simulink model "C_H_B - Copy"  (R2017a)
settings: Solver=ode23t  StartTime=0.0  StopTime=0.08  FixedStep=5e-5  MaxStep=1e-4  RelTol=1e-3
undefined symbols (not defined in the file): a1, a2, a3, Vdc
libraries: powerlib x50, simulink x6
settings Model: Creator=Vinay  LastModifiedBy=murra

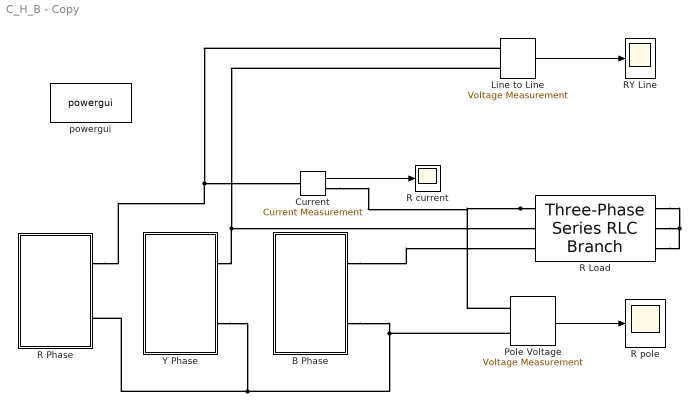
== system C_H_B - Copy ==
  B Phase : Subsystem
  Current : powerlib/Measurements/Current Measurement  PhasorSimulation=off  OutputType=Complex  PSBequivalent=0
  Line to Line : powerlib/Measurements/Voltage Measurement  PhasorSimulation=off  OutputType=Complex  PSBequivalent=0
  "Pole Voltage  " : powerlib/Measurements/Voltage Measurement  PhasorSimulation=off  OutputType=Complex  PSBequivalent=0
  R Load : powerlib/Elements/Three-Phase Series RLC Branch  LConnTagsString=A|B|C  RConnTagsString=A|B|C  BranchType=RL  Resistance=100  Inductance=1.5e-3  Capacitance=1e-6  Measurements=None
  R Phase : Subsystem
  R current : Scope
  R pole : Scope
  RY Line : Scope
  Y Phase : Subsystem
  powergui : powerlib/powergui  Priority=1  SimulationMode=Discrete  SampleTime=1e-06  frequency=60  Iterations=50  frequencyindice=0  Pbase=100e6  ErrMax=1e-4  UnitsV=kV  UnitsW=MW  buscounter=0  FunctionMessages=off  echomessages=off  EnableUseOfTLC=off  CurrentSourceSwitches=off  DisableSnubberDevices=off  DisableRonSwitches=off  DisableVfSwitches=off  DisplayEquations=off  SolverType=Tustin/Backward Euler (TBE)  Interpol=off  ExternalGateDelay=off  methode=off  Ts=100  x0status=blocks  SPID=on  SwTol=0  HookPort=off  RestoreLinks=warning  ResistiveCurrentMeasurement=off  Frange=[0:2:500]  Ylog=off  Xlog=on  ShowGrid=off  save=off  variable=ZData  structure=Rpole  ZoomFFT=off  StartTime=0.02  cycles=2  DisplayStyle=2  fundamental=50  FreqAxis=off  MaxFrequency=10000  frequencyindicesteady=1  RmsSteady=1  display=off
  wires:
  Line to Line/1 -> RY Line/1
  "Pole Voltage  "/1 -> R pole/1
  Current/1 -> R current/1
  connections:
  B Phase/RConn2 -- "Pole Voltage  "/LConn2 -- Y Phase/RConn2 -- R Phase/RConn2
  R Phase/RConn1 -- Line to Line/LConn1 -- Current/LConn1
  Y Phase/RConn1 -- Line to Line/LConn2 -- R Load/LConn2
  B Phase/RConn1 -- R Load/LConn3
  R Load/RConn3 -- R Load/RConn1 -- R Load/RConn2
  R Load/LConn1 -- "Pole Voltage  "/LConn1 -- Current/RConn1

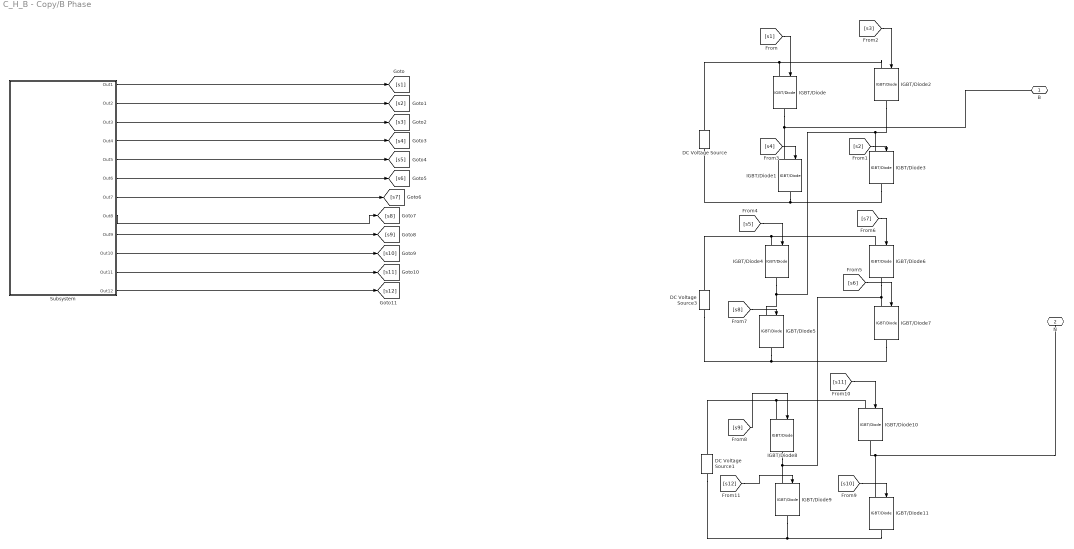
== system C_H_B - Copy/B Phase ==
  DC Voltage Source : powerlib/Electrical Sources/DC Voltage Source  Amplitude=Vdc  Measurements=None
  DC Voltage Source1 : powerlib/Electrical Sources/DC Voltage Source  Amplitude=Vdc  Measurements=None
  DC Voltage Source3 : powerlib/Electrical Sources/DC Voltage Source  Amplitude=Vdc  Measurements=None
  IGBT/Diode{,1..11} (12 alike) : powerlib/Power Electronics/IGBT//Diode  Ron=1e-3  Rs=1e5  Cs=inf  Measurements=off
  Subsystem : Subsystem
  B : PMIOPort  Port=1  Side=Right
  N : PMIOPort  Port=2  Side=Right
  wires:
  [s3] -> IGBT/Diode2/1
  [s6] -> IGBT/Diode7/1
  [s4] -> IGBT/Diode1/1
  [s8] -> IGBT/Diode5/1
  [s12] -> IGBT/Diode9/1
  [s2] -> IGBT/Diode3/1
  [s7] -> IGBT/Diode6/1
  [s9] -> IGBT/Diode8/1
  [s1] -> IGBT/Diode/1
  [s10] -> IGBT/Diode11/1
  [s5] -> IGBT/Diode4/1
  [s11] -> IGBT/Diode10/1
  Subsystem/5(Out5) -> [s5]
  Subsystem/7(Out7) -> [s7]
  Subsystem/8(Out8) -> [s8]
  Subsystem/3(Out3) -> [s3]
  Subsystem/10(Out10) -> [s10]
  Subsystem/1(Out1) -> [s1]
  Subsystem/11(Out11) -> [s11]
  Subsystem/2(Out2) -> [s2]
  Subsystem/12(Out12) -> [s12]
  Subsystem/6(Out6) -> [s6]
  Subsystem/9(Out9) -> [s9]
  Subsystem/4(Out4) -> [s4]
  connections:
  IGBT/Diode10/RConn1 -- IGBT/Diode11/LConn1 -- N/RConn1
  DC Voltage Source1/LConn1 -- IGBT/Diode11/RConn1 -- IGBT/Diode9/RConn1
  DC Voltage Source3/RConn1 -- IGBT/Diode6/LConn1 -- IGBT/Diode4/LConn1
  DC Voltage Source1/RConn1 -- IGBT/Diode10/LConn1 -- IGBT/Diode8/LConn1
  DC Voltage Source/RConn1 -- IGBT/Diode2/LConn1 -- IGBT/Diode/LConn1
  DC Voltage Source3/LConn1 -- IGBT/Diode7/RConn1 -- IGBT/Diode5/RConn1
  IGBT/Diode/RConn1 -- IGBT/Diode1/LConn1 -- B/RConn1
  IGBT/Diode9/LConn1 -- IGBT/Diode8/RConn1 -- IGBT/Diode7/LConn1 -- IGBT/Diode6/RConn1
  IGBT/Diode3/LConn1 -- IGBT/Diode2/RConn1 -- IGBT/Diode5/LConn1 -- IGBT/Diode4/RConn1
  DC Voltage Source/LConn1 -- IGBT/Diode1/RConn1 -- IGBT/Diode3/RConn1

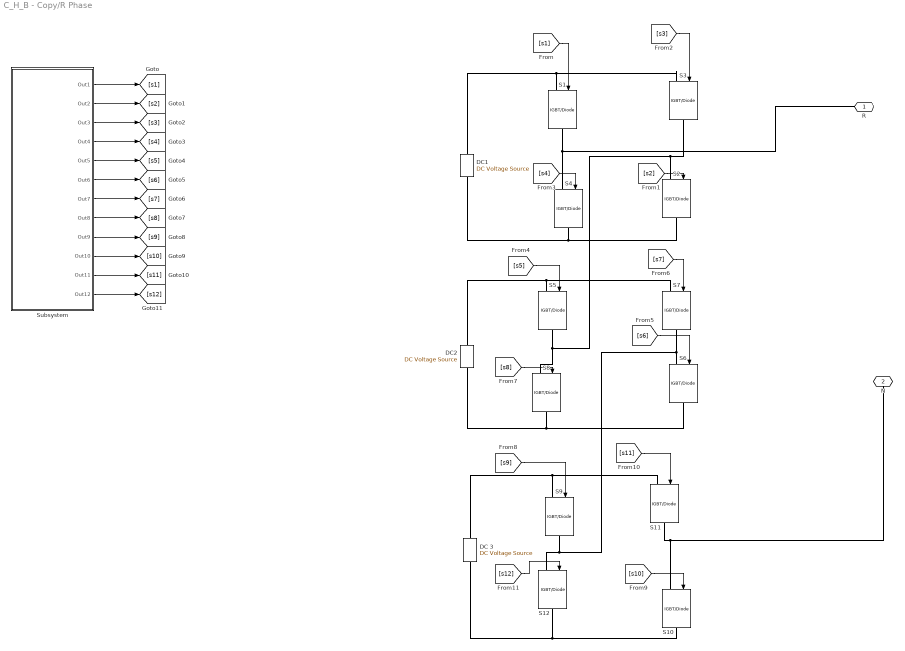
== system C_H_B - Copy/R Phase ==
  DC 3 : powerlib/Electrical Sources/DC Voltage Source  Amplitude=Vdc  Measurements=None
  DC1 : powerlib/Electrical Sources/DC Voltage Source  Amplitude=Vdc  Measurements=None
  DC2 : powerlib/Electrical Sources/DC Voltage Source  Amplitude=Vdc  Measurements=None
  S{1..12} (12 alike) : powerlib/Power Electronics/IGBT//Diode  Ron=1e-3  Rs=1e5  Cs=inf  Measurements=off
  Subsystem : Subsystem
  R : PMIOPort  Port=1  Side=Right
  N : PMIOPort  Port=2  Side=Right
  wires:
  [s3] -> S3/1
  [s6] -> S6/1
  [s4] -> S4/1
  [s8] -> S8/1
  [s12] -> S12/1
  [s2] -> S2/1
  [s7] -> S7/1
  [s9] -> S9/1
  [s1] -> S1/1
  [s10] -> S10/1
  [s5] -> S5/1
  [s11] -> S11/1
  Subsystem/5(Out5) -> [s5]
  Subsystem/7(Out7) -> [s7]
  Subsystem/8(Out8) -> [s8]
  Subsystem/3(Out3) -> [s3]
  Subsystem/10(Out10) -> [s10]
  Subsystem/1(Out1) -> [s1]
  Subsystem/11(Out11) -> [s11]
  Subsystem/2(Out2) -> [s2]
  Subsystem/12(Out12) -> [s12]
  Subsystem/6(Out6) -> [s6]
  Subsystem/9(Out9) -> [s9]
  Subsystem/4(Out4) -> [s4]
  connections:
  S11/RConn1 -- N/RConn1 -- S10/LConn1
  DC 3/LConn1 -- S10/RConn1 -- S12/RConn1
  DC2/RConn1 -- S7/LConn1 -- S5/LConn1
  DC 3/RConn1 -- S11/LConn1 -- S9/LConn1
  DC1/RConn1 -- S3/LConn1 -- S1/LConn1
  DC2/LConn1 -- S6/RConn1 -- S8/RConn1
  S1/RConn1 -- R/RConn1 -- S4/LConn1
  S12/LConn1 -- S9/RConn1 -- S6/LConn1 -- S7/RConn1
  S2/LConn1 -- S3/RConn1 -- S8/LConn1 -- S5/RConn1
  DC1/LConn1 -- S4/RConn1 -- S2/RConn1

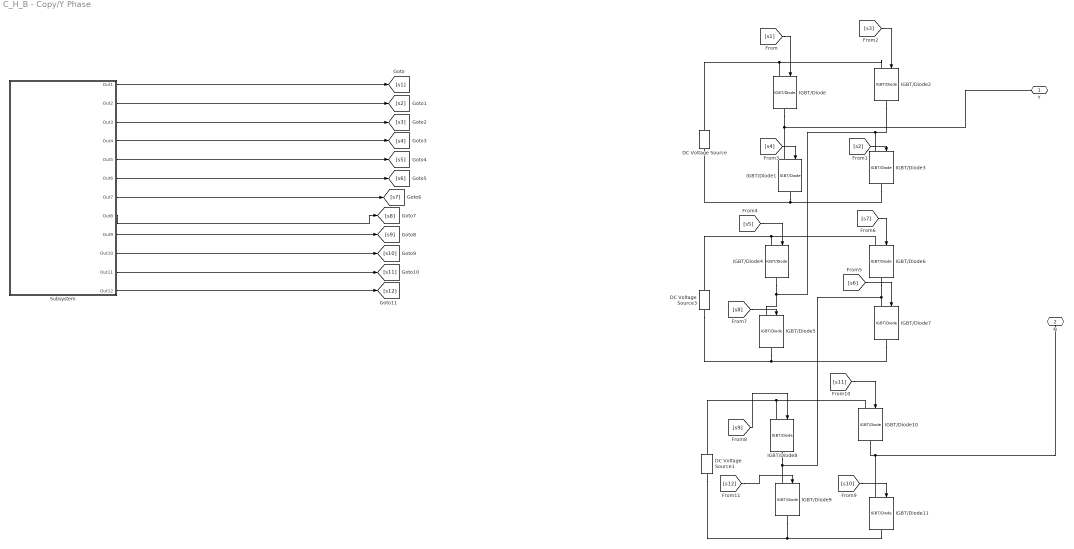
== system C_H_B - Copy/Y Phase ==
  DC Voltage Source : powerlib/Electrical Sources/DC Voltage Source  Amplitude=Vdc  Measurements=None
  DC Voltage Source1 : powerlib/Electrical Sources/DC Voltage Source  Amplitude=Vdc  Measurements=None
  DC Voltage Source3 : powerlib/Electrical Sources/DC Voltage Source  Amplitude=Vdc  Measurements=None
  IGBT/Diode{,1..11} (12 alike) : powerlib/Power Electronics/IGBT//Diode  Ron=1e-3  Rs=1e5  Cs=inf  Measurements=off
  Subsystem : Subsystem
  Y : PMIOPort  Port=1  Side=Right
  N : PMIOPort  Port=2  Side=Right
  wires:
  [s3] -> IGBT/Diode2/1
  [s6] -> IGBT/Diode7/1
  [s4] -> IGBT/Diode1/1
  [s8] -> IGBT/Diode5/1
  [s12] -> IGBT/Diode9/1
  [s2] -> IGBT/Diode3/1
  [s7] -> IGBT/Diode6/1
  [s9] -> IGBT/Diode8/1
  [s1] -> IGBT/Diode/1
  [s10] -> IGBT/Diode11/1
  [s5] -> IGBT/Diode4/1
  [s11] -> IGBT/Diode10/1
  Subsystem/5(Out5) -> [s5]
  Subsystem/7(Out7) -> [s7]
  Subsystem/8(Out8) -> [s8]
  Subsystem/3(Out3) -> [s3]
  Subsystem/10(Out10) -> [s10]
  Subsystem/1(Out1) -> [s1]
  Subsystem/11(Out11) -> [s11]
  Subsystem/2(Out2) -> [s2]
  Subsystem/12(Out12) -> [s12]
  Subsystem/6(Out6) -> [s6]
  Subsystem/9(Out9) -> [s9]
  Subsystem/4(Out4) -> [s4]
  connections:
  IGBT/Diode10/RConn1 -- IGBT/Diode11/LConn1 -- N/RConn1
  DC Voltage Source1/LConn1 -- IGBT/Diode11/RConn1 -- IGBT/Diode9/RConn1
  DC Voltage Source3/RConn1 -- IGBT/Diode6/LConn1 -- IGBT/Diode4/LConn1
  DC Voltage Source1/RConn1 -- IGBT/Diode10/LConn1 -- IGBT/Diode8/LConn1
  DC Voltage Source/RConn1 -- IGBT/Diode2/LConn1 -- IGBT/Diode/LConn1
  DC Voltage Source3/LConn1 -- IGBT/Diode7/RConn1 -- IGBT/Diode5/RConn1
  IGBT/Diode/RConn1 -- IGBT/Diode1/LConn1 -- Y/RConn1
  IGBT/Diode9/LConn1 -- IGBT/Diode8/RConn1 -- IGBT/Diode7/LConn1 -- IGBT/Diode6/RConn1
  IGBT/Diode3/LConn1 -- IGBT/Diode2/RConn1 -- IGBT/Diode5/LConn1 -- IGBT/Diode4/RConn1
  DC Voltage Source/LConn1 -- IGBT/Diode1/RConn1 -- IGBT/Diode3/RConn1

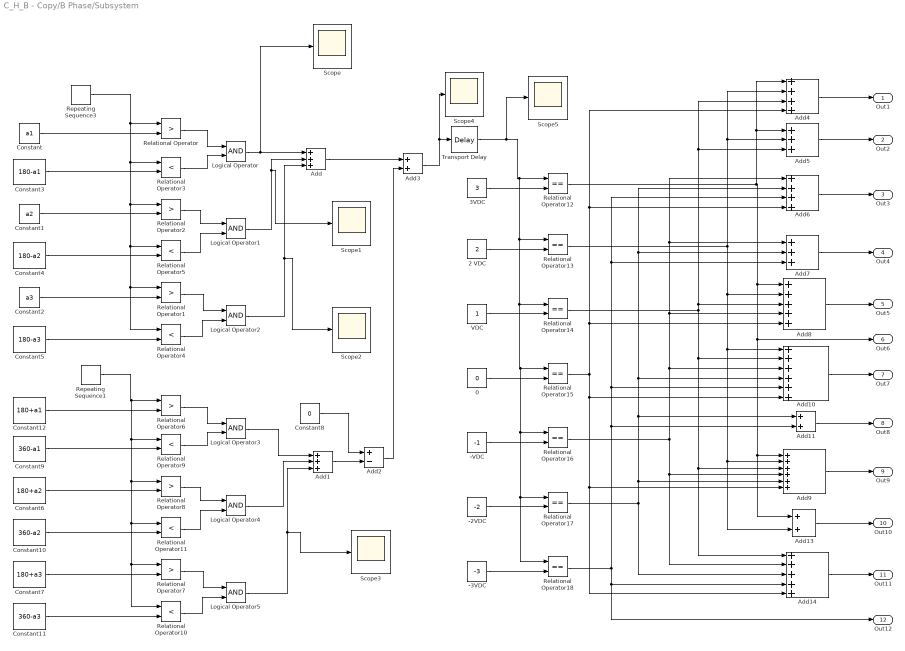
== system C_H_B - Copy/B Phase/Subsystem ==
  -2VDC : Constant  Value=-2
  -3VDC : Constant  Value=-3
  -VDC : Constant  Value=-1
  0 : Constant  Value=0
  2 VDC : Constant  Value=2
  3VDC : Constant  Value=3
  Add{,1,5,7} (4 alike) : Sum  Inputs=+++
  Add10 : Sum  Inputs=++++++
  Add11 : Sum
  Add13 : Sum
  Add14 : Sum  Inputs=+++++
  Add2 : Sum  Inputs=+-
  Add3 : Sum
  Add4 : Sum  Inputs=++++
  Add6 : Sum  Inputs=++++
  Add8 : Sum  Inputs=+++++
  Add9 : Sum  Inputs=++++++
  Constant : Constant  Value=a1
  Constant1 : Constant  Value=a2
  Constant10 : Constant  Value=360-a2
  Constant11 : Constant  Value=360-a3
  Constant12 : Constant  Value=180+a1
  Constant2 : Constant  Value=a3
  Constant3 : Constant  Value=180-a1
  Constant4 : Constant  Value=180-a2
  Constant5 : Constant  Value=180-a3
  Constant6 : Constant  Value=180+a2
  Constant7 : Constant  Value=180+a3
  Constant8 : Constant  Value=0
  Constant9 : Constant  Value=360-a1
  Logical Operator{,1..5} (6 alike) : Logic  AllPortsSameDT=off  OutDataTypeStr=boolean
  Relational Operator{,1..2,6..8} (6 alike) : RelationalOperator  Operator=>  OutDataTypeStr=boolean  RndMeth=Simplest
  Relational Operator{3..5,9..11} (6 alike) : RelationalOperator  Operator=<  OutDataTypeStr=boolean  RndMeth=Simplest
  Relational Operator{12..18} (7 alike) : RelationalOperator  Operator===  OutDataTypeStr=boolean  RndMeth=Simplest
  Repeating Sequence1 : simulink/Sources/Repeating Sequence  rep_seq_t=[0 0.02]  rep_seq_y=[0 360]
  Repeating Sequence3 : simulink/Sources/Repeating Sequence  rep_seq_t=[0 0.02]  rep_seq_y=[0 360]
  Scope{,1..5} (6 alike) : Scope
  Transport Delay : TransportDelay  DelayTime=0.04/3  BufferSize=30000
  VDC : Constant
  Out1 : Outport
  Out2 : Outport  Port=2
  Out3 : Outport  Port=3
  Out4 : Outport  Port=4
  Out5 : Outport  Port=5
  Out6 : Outport  Port=6
  Out7 : Outport  Port=7
  Out8 : Outport  Port=8
  Out9 : Outport  Port=9
  Out10 : Outport  Port=10
  Out11 : Outport  Port=11
  Out12 : Outport  Port=12
  wires:
  Logical Operator2/1 -> Scope2/1, Add/3
  Constant/1 -> Relational Operator/2
  -2VDC/1 -> Relational Operator17/2
  Add13/1 -> Out10/1
  Add3/1 -> Scope4/1, Transport Delay/1
  Relational Operator/1 -> Logical Operator/1
  Relational Operator15/1 -> Add6/4, Add4/4, Add8/5, Add14/5, Add9/6, Add10/6
  Repeating Sequence3/1 -> Relational Operator3/1, Relational Operator2/1, Relational Operator1/1, Relational Operator4/1, Relational Operator5/1, Relational Operator/1
  Relational Operator18/1 -> Out12/1, Add14/4, Add11/2, Add10/5, Add7/3, Add6/3
  Constant6/1 -> Relational Operator8/2
  Add5/1 -> Out2/1
  Add/1 -> Add3/1
  Constant2/1 -> Relational Operator1/2
  Add2/1 -> Add3/2
  Relational Operator8/1 -> Logical Operator4/1
  Repeating Sequence1/1 -> Relational Operator8/1, Relational Operator11/1, Relational Operator10/1, Relational Operator7/1, Relational Operator9/1, Relational Operator6/1
  Relational Operator9/1 -> Logical Operator3/2
  Relational Operator13/1 -> Add13/2, Add9/2, Add10/1, Add8/2, Add5/2, Add4/2
  0/1 -> Relational Operator15/2
  Constant3/1 -> Relational Operator3/2
  Relational Operator3/1 -> Logical Operator/2
  Relational Operator5/1 -> Logical Operator1/2
  Add1/1 -> Add2/2
  Logical Operator/1 -> Scope/1, Add/1
  Relational Operator1/1 -> Logical Operator2/1
  Add9/1 -> Out9/1
  Logical Operator5/1 -> Scope3/1, Add1/3
  Logical Operator1/1 -> Scope1/1, Add/2
  Relational Operator12/1 -> Add5/1, Add4/1, Out6/1, Add13/1, Add9/1, Add8/1
  Relational Operator4/1 -> Logical Operator2/2
  Relational Operator11/1 -> Logical Operator4/2
  Relational Operator2/1 -> Logical Operator1/1
  Relational Operator16/1 -> Add10/3, Add8/4, Add7/1, Add6/1, Add14/2, Add9/4
  Constant5/1 -> Relational Operator4/2
  Constant1/1 -> Relational Operator2/2
  Constant7/1 -> Relational Operator7/2
  Constant4/1 -> Relational Operator5/2
  Constant12/1 -> Relational Operator6/2
  Add10/1 -> Out7/1
  Add8/1 -> Out5/1
  -VDC/1 -> Relational Operator16/2
  Relational Operator17/1 -> Add14/3, Add9/5, Add11/1, Add10/4, Add7/2, Add6/2
  Add6/1 -> Out3/1
  3VDC/1 -> Relational Operator12/2
  Constant11/1 -> Relational Operator10/2
  Logical Operator3/1 -> Add1/1
  VDC/1 -> Relational Operator14/2
  Constant9/1 -> Relational Operator9/2
  Add4/1 -> Out1/1
  Relational Operator7/1 -> Logical Operator5/1
  Add11/1 -> Out8/1
  Logical Operator4/1 -> Add1/2
  -3VDC/1 -> Relational Operator18/2
  Constant8/1 -> Add2/1
  Add14/1 -> Out11/1
  2 VDC/1 -> Relational Operator13/2
  Constant10/1 -> Relational Operator11/2
  Relational Operator14/1 -> Add14/1, Add9/3, Add10/2, Add5/3, Add4/3, Add8/3
  Add7/1 -> Out4/1
  Relational Operator10/1 -> Logical Operator5/2
  Relational Operator6/1 -> Logical Operator3/1
  Transport Delay/1 -> Scope5/1, Relational Operator18/1, Relational Operator17/1, Relational Operator16/1, Relational Operator15/1, Relational Operator14/1, Relational Operator13/1, Relational Operator12/1

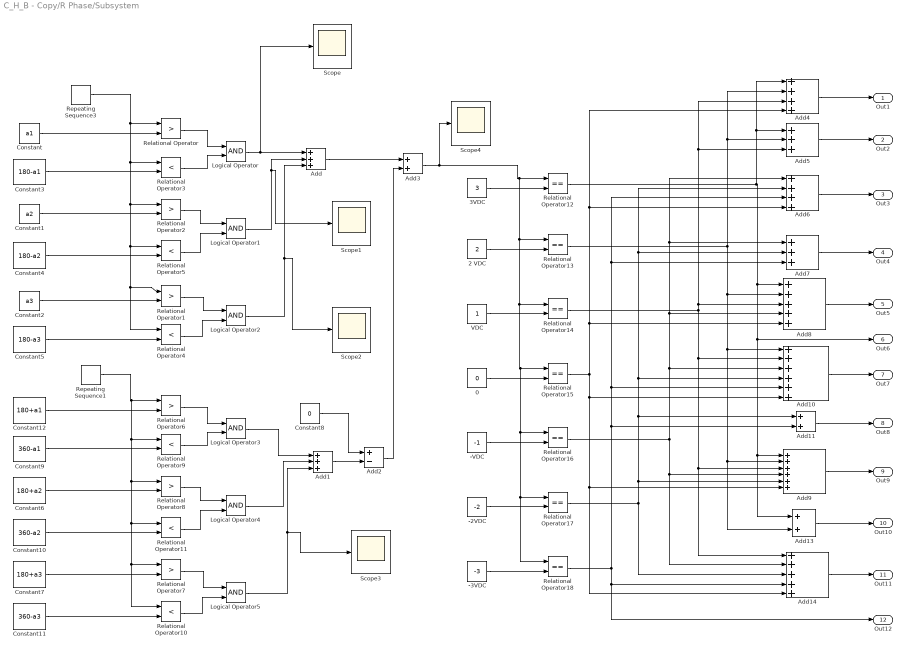
== system C_H_B - Copy/R Phase/Subsystem ==
  -2VDC : Constant  Value=-2
  -3VDC : Constant  Value=-3
  -VDC : Constant  Value=-1
  0 : Constant  Value=0
  2 VDC : Constant  Value=2
  3VDC : Constant  Value=3
  Add{,1,5,7} (4 alike) : Sum  Inputs=+++
  Add10 : Sum  Inputs=++++++
  Add11 : Sum
  Add13 : Sum
  Add14 : Sum  Inputs=+++++
  Add2 : Sum  Inputs=+-
  Add3 : Sum
  Add4 : Sum  Inputs=++++
  Add6 : Sum  Inputs=++++
  Add8 : Sum  Inputs=+++++
  Add9 : Sum  Inputs=++++++
  Constant : Constant  Value=a1
  Constant1 : Constant  Value=a2
  Constant10 : Constant  Value=360-a2
  Constant11 : Constant  Value=360-a3
  Constant12 : Constant  Value=180+a1
  Constant2 : Constant  Value=a3
  Constant3 : Constant  Value=180-a1
  Constant4 : Constant  Value=180-a2
  Constant5 : Constant  Value=180-a3
  Constant6 : Constant  Value=180+a2
  Constant7 : Constant  Value=180+a3
  Constant8 : Constant  Value=0
  Constant9 : Constant  Value=360-a1
  Logical Operator{,1..5} (6 alike) : Logic  AllPortsSameDT=off  OutDataTypeStr=boolean
  Relational Operator{,1..2,6..8} (6 alike) : RelationalOperator  Operator=>  OutDataTypeStr=boolean  RndMeth=Simplest
  Relational Operator{3..5,9..11} (6 alike) : RelationalOperator  Operator=<  OutDataTypeStr=boolean  RndMeth=Simplest
  Relational Operator{12..18} (7 alike) : RelationalOperator  Operator===  OutDataTypeStr=boolean  RndMeth=Simplest
  Repeating Sequence1 : simulink/Sources/Repeating Sequence  rep_seq_t=[0 0.02]  rep_seq_y=[0 360]
  Repeating Sequence3 : simulink/Sources/Repeating Sequence  rep_seq_t=[0 0.02]  rep_seq_y=[0 360]
  Scope{,1..4} (5 alike) : Scope
  VDC : Constant
  Out1 : Outport
  Out2 : Outport  Port=2
  Out3 : Outport  Port=3
  Out4 : Outport  Port=4
  Out5 : Outport  Port=5
  Out6 : Outport  Port=6
  Out7 : Outport  Port=7
  Out8 : Outport  Port=8
  Out9 : Outport  Port=9
  Out10 : Outport  Port=10
  Out11 : Outport  Port=11
  Out12 : Outport  Port=12
  wires:
  Logical Operator2/1 -> Scope2/1, Add/3
  Constant/1 -> Relational Operator/2
  -2VDC/1 -> Relational Operator17/2
  Add13/1 -> Out10/1
  Add3/1 -> Scope4/1, Relational Operator18/1, Relational Operator17/1, Relational Operator16/1, Relational Operator15/1, Relational Operator14/1, Relational Operator13/1, Relational Operator12/1
  Relational Operator/1 -> Logical Operator/1
  Relational Operator15/1 -> Add6/4, Add4/4, Add8/5, Add14/5, Add9/6, Add10/6
  Repeating Sequence3/1 -> Relational Operator3/1, Relational Operator2/1, Relational Operator1/1, Relational Operator4/1, Relational Operator5/1, Relational Operator/1
  Relational Operator18/1 -> Out12/1, Add14/4, Add11/2, Add10/5, Add7/3, Add6/3
  Constant6/1 -> Relational Operator8/2
  Add5/1 -> Out2/1
  Add/1 -> Add3/1
  Add2/1 -> Add3/2
  Relational Operator8/1 -> Logical Operator4/1
  Repeating Sequence1/1 -> Relational Operator8/1, Relational Operator11/1, Relational Operator10/1, Relational Operator7/1, Relational Operator9/1, Relational Operator6/1
  Relational Operator9/1 -> Logical Operator3/2
  Relational Operator13/1 -> Add13/2, Add9/2, Add10/1, Add8/2, Add5/2, Add4/2
  0/1 -> Relational Operator15/2
  Constant3/1 -> Relational Operator3/2
  Relational Operator3/1 -> Logical Operator/2
  Relational Operator5/1 -> Logical Operator1/2
  Add1/1 -> Add2/2
  Logical Operator/1 -> Scope/1, Add/1
  Relational Operator1/1 -> Logical Operator2/1
  Add9/1 -> Out9/1
  Logical Operator5/1 -> Scope3/1, Add1/3
  Logical Operator1/1 -> Scope1/1, Add/2
  Relational Operator12/1 -> Add5/1, Add4/1, Out6/1, Add13/1, Add9/1, Add8/1
  Relational Operator4/1 -> Logical Operator2/2
  Relational Operator11/1 -> Logical Operator4/2
  Relational Operator2/1 -> Logical Operator1/1
  Relational Operator16/1 -> Add10/3, Add8/4, Add7/1, Add6/1, Add14/2, Add9/4
  Constant5/1 -> Relational Operator4/2
  Constant1/1 -> Relational Operator2/2
  Constant7/1 -> Relational Operator7/2
  Constant4/1 -> Relational Operator5/2
  Constant12/1 -> Relational Operator6/2
  Add10/1 -> Out7/1
  Add8/1 -> Out5/1
  -VDC/1 -> Relational Operator16/2
  Relational Operator17/1 -> Add14/3, Add9/5, Add11/1, Add10/4, Add7/2, Add6/2
  Add6/1 -> Out3/1
  3VDC/1 -> Relational Operator12/2
  Constant11/1 -> Relational Operator10/2
  Logical Operator3/1 -> Add1/1
  VDC/1 -> Relational Operator14/2
  Constant9/1 -> Relational Operator9/2
  Add4/1 -> Out1/1
  Relational Operator7/1 -> Logical Operator5/1
  Add11/1 -> Out8/1
  Logical Operator4/1 -> Add1/2
  -3VDC/1 -> Relational Operator18/2
  Constant8/1 -> Add2/1
  Add14/1 -> Out11/1
  2 VDC/1 -> Relational Operator13/2
  Constant10/1 -> Relational Operator11/2
  Relational Operator14/1 -> Add14/1, Add9/3, Add10/2, Add5/3, Add4/3, Add8/3
  Add7/1 -> Out4/1
  Relational Operator10/1 -> Logical Operator5/2
  Relational Operator6/1 -> Logical Operator3/1
  Constant2/1 -> Relational Operator1/2

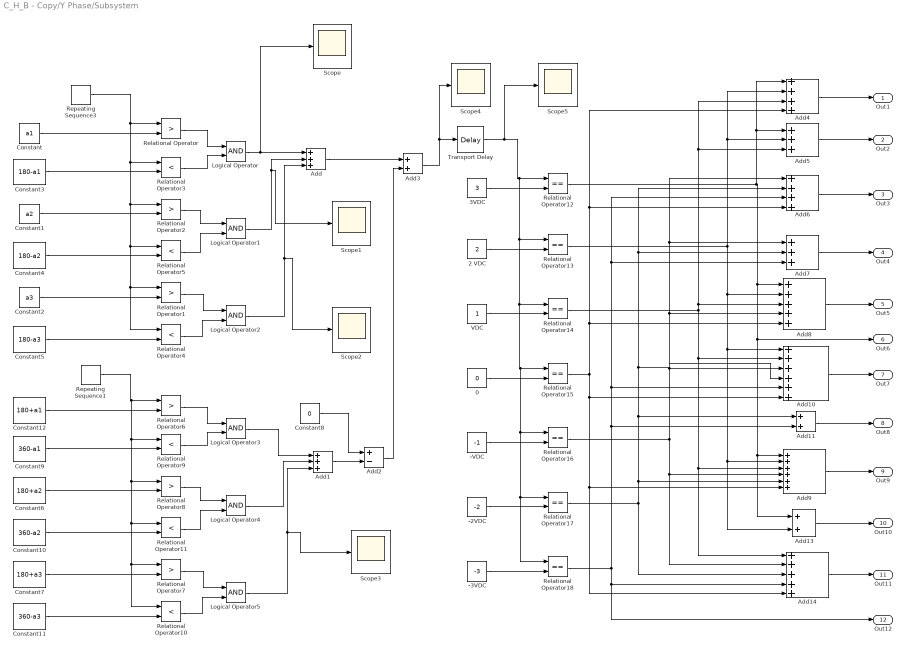
== system C_H_B - Copy/Y Phase/Subsystem ==
  -2VDC : Constant  Value=-2
  -3VDC : Constant  Value=-3
  -VDC : Constant  Value=-1
  0 : Constant  Value=0
  2 VDC : Constant  Value=2
  3VDC : Constant  Value=3
  Add{,1,5,7} (4 alike) : Sum  Inputs=+++
  Add10 : Sum  Inputs=++++++
  Add11 : Sum
  Add13 : Sum
  Add14 : Sum  Inputs=+++++
  Add2 : Sum  Inputs=+-
  Add3 : Sum
  Add4 : Sum  Inputs=++++
  Add6 : Sum  Inputs=++++
  Add8 : Sum  Inputs=+++++
  Add9 : Sum  Inputs=++++++
  Constant : Constant  Value=a1
  Constant1 : Constant  Value=a2
  Constant10 : Constant  Value=360-a2
  Constant11 : Constant  Value=360-a3
  Constant12 : Constant  Value=180+a1
  Constant2 : Constant  Value=a3
  Constant3 : Constant  Value=180-a1
  Constant4 : Constant  Value=180-a2
  Constant5 : Constant  Value=180-a3
  Constant6 : Constant  Value=180+a2
  Constant7 : Constant  Value=180+a3
  Constant8 : Constant  Value=0
  Constant9 : Constant  Value=360-a1
  Logical Operator{,1..5} (6 alike) : Logic  AllPortsSameDT=off  OutDataTypeStr=boolean
  Relational Operator{,1..2,6..8} (6 alike) : RelationalOperator  Operator=>  OutDataTypeStr=boolean  RndMeth=Simplest
  Relational Operator{3..5,9..11} (6 alike) : RelationalOperator  Operator=<  OutDataTypeStr=boolean  RndMeth=Simplest
  Relational Operator{12..18} (7 alike) : RelationalOperator  Operator===  OutDataTypeStr=boolean  RndMeth=Simplest
  Repeating Sequence1 : simulink/Sources/Repeating Sequence  rep_seq_t=[0 0.02]  rep_seq_y=[0 360]
  Repeating Sequence3 : simulink/Sources/Repeating Sequence  rep_seq_t=[0 0.02]  rep_seq_y=[0 360]
  Scope{,1..5} (6 alike) : Scope
  Transport Delay : TransportDelay  DelayTime=0.02/3  BufferSize=30000
  VDC : Constant
  Out1 : Outport
  Out2 : Outport  Port=2
  Out3 : Outport  Port=3
  Out4 : Outport  Port=4
  Out5 : Outport  Port=5
  Out6 : Outport  Port=6
  Out7 : Outport  Port=7
  Out8 : Outport  Port=8
  Out9 : Outport  Port=9
  Out10 : Outport  Port=10
  Out11 : Outport  Port=11
  Out12 : Outport  Port=12
  wires:
  Logical Operator2/1 -> Scope2/1, Add/3
  Constant/1 -> Relational Operator/2
  -2VDC/1 -> Relational Operator17/2
  Add13/1 -> Out10/1
  Add3/1 -> Scope4/1, Transport Delay/1
  Relational Operator/1 -> Logical Operator/1
  Relational Operator15/1 -> Add6/4, Add4/4, Add8/5, Add14/5, Add9/6, Add10/6
  Repeating Sequence3/1 -> Relational Operator3/1, Relational Operator2/1, Relational Operator1/1, Relational Operator4/1, Relational Operator5/1, Relational Operator/1
  Relational Operator18/1 -> Out12/1, Add14/4, Add11/2, Add10/5, Add7/3, Add6/3
  Constant6/1 -> Relational Operator8/2
  Add5/1 -> Out2/1
  Add/1 -> Add3/1
  Constant2/1 -> Relational Operator1/2
  Add2/1 -> Add3/2
  Relational Operator8/1 -> Logical Operator4/1
  Repeating Sequence1/1 -> Relational Operator8/1, Relational Operator11/1, Relational Operator10/1, Relational Operator7/1, Relational Operator9/1, Relational Operator6/1
  Relational Operator9/1 -> Logical Operator3/2
  Relational Operator13/1 -> Add13/2, Add9/2, Add10/1, Add8/2, Add5/2, Add4/2
  0/1 -> Relational Operator15/2
  Constant3/1 -> Relational Operator3/2
  Relational Operator3/1 -> Logical Operator/2
  Relational Operator5/1 -> Logical Operator1/2
  Add1/1 -> Add2/2
  Logical Operator/1 -> Scope/1, Add/1
  Relational Operator1/1 -> Logical Operator2/1
  Add9/1 -> Out9/1
  Logical Operator5/1 -> Scope3/1, Add1/3
  Logical Operator1/1 -> Scope1/1, Add/2
  Relational Operator12/1 -> Add5/1, Add4/1, Out6/1, Add13/1, Add9/1, Add8/1
  Relational Operator4/1 -> Logical Operator2/2
  Relational Operator11/1 -> Logical Operator4/2
  Relational Operator2/1 -> Logical Operator1/1
  Relational Operator16/1 -> Add10/3, Add8/4, Add7/1, Add6/1, Add14/2, Add9/4
  Constant5/1 -> Relational Operator4/2
  Constant1/1 -> Relational Operator2/2
  Constant7/1 -> Relational Operator7/2
  Constant4/1 -> Relational Operator5/2
  Constant12/1 -> Relational Operator6/2
  Add10/1 -> Out7/1
  Add8/1 -> Out5/1
  -VDC/1 -> Relational Operator16/2
  Relational Operator17/1 -> Add14/3, Add9/5, Add11/1, Add10/4, Add7/2, Add6/2
  Add6/1 -> Out3/1
  3VDC/1 -> Relational Operator12/2
  Constant11/1 -> Relational Operator10/2
  Logical Operator3/1 -> Add1/1
  VDC/1 -> Relational Operator14/2
  Constant9/1 -> Relational Operator9/2
  Add4/1 -> Out1/1
  Relational Operator7/1 -> Logical Operator5/1
  Add11/1 -> Out8/1
  Logical Operator4/1 -> Add1/2
  -3VDC/1 -> Relational Operator18/2
  Constant8/1 -> Add2/1
  Add14/1 -> Out11/1
  2 VDC/1 -> Relational Operator13/2
  Constant10/1 -> Relational Operator11/2
  Relational Operator14/1 -> Add14/1, Add9/3, Add10/2, Add5/3, Add4/3, Add8/3
  Add7/1 -> Out4/1
  Relational Operator10/1 -> Logical Operator5/2
  Relational Operator6/1 -> Logical Operator3/1
  Transport Delay/1 -> Scope5/1, Relational Operator18/1, Relational Operator17/1, Relational Operator16/1, Relational Operator15/1, Relational Operator14/1, Relational Operator13/1, Relational Operator12/1
